simulink model "Uklad_Obiekt_Regulator_Calka150"  (R2024a)
settings: Solver=VariableStepAuto  StartTime=0.0  StopTime=10.0  RelTol=1e-3
values from neighbouring files (symbols this model uses):
  K = K_r(1:end-1)    [oblicz_parametry_obserwatora_z_calkowaniem.m]    (also in oblicz_parametry_regulatora.m = acker(A, B, [s_b s_b s_b]); symulacjeObserwator.m = oblicz_parametry_regulatora(A, B, s_b); symulacjeObserwatorZero.m = oblicz_parametry_regulatora(A, B, s_b); symulacjeRegulator.m = oblicz_parametry_regulatora(A, B, s_b))
  K_e = K_r(end)    [oblicz_parametry_obserwatora_z_calkowaniem.m]
  X_0 = [1; -5; 1]    [symulacjeObserwator.m]    (also in symulacjeObserwatorZero.m; symulacjeRegulator.m; symulacjeRegulatorCalka.m = [0; 0; 0]; symulacjeRegulatorCalka150.m = [0; 0; 0])
  y_zad = 10    [symulacjeRegulatorCalka.m]    (also in symulacjeRegulatorCalka150.m)
settings Model: Creator=pioro  LastModifiedBy=pioro

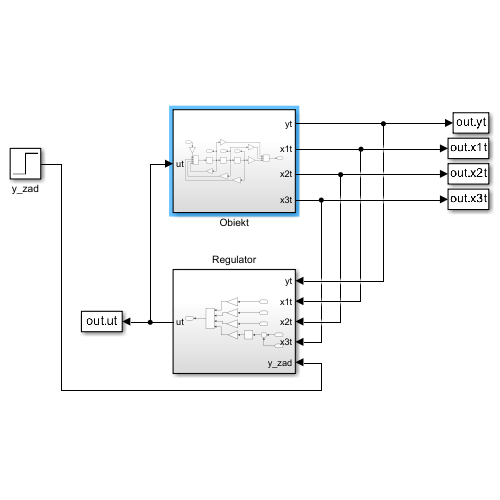
[thumbnail: Simulink's stored preview of the top-level diagram]
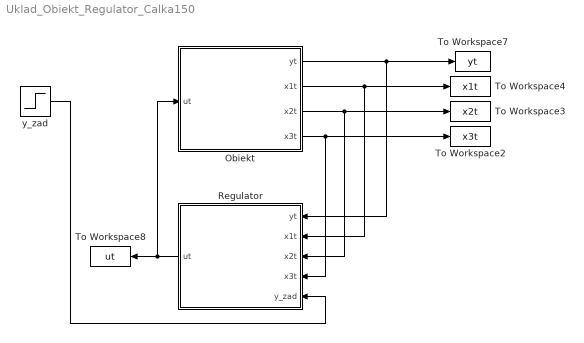
== system Uklad_Obiekt_Regulator_Calka150 ==
  Obiekt : Subsystem
  Regulator : Subsystem
  To Workspace2 : ToWorkspace  VariableName=x3t  SaveFormat=Timeseries  SampleTime=-1
  To Workspace3 : ToWorkspace  VariableName=x2t  SaveFormat=Timeseries  SampleTime=-1
  To Workspace4 : ToWorkspace  VariableName=x1t  SaveFormat=Timeseries  SampleTime=-1
  To Workspace7 : ToWorkspace  VariableName=yt  SaveFormat=Timeseries  SampleTime=-1
  To Workspace8 : ToWorkspace  VariableName=ut  SaveFormat=Timeseries  SampleTime=-1
  y_zad : Step  After=y_zad  SampleTime=0
  wires:
  Obiekt/3(x2t) -> To Workspace3/1, Regulator/3(x2t)
  y_zad/1 -> Regulator/5(y_zad)
  Obiekt/1(yt) -> Regulator/1(yt), To Workspace7/1
  Regulator/1(ut) -> Obiekt/1(ut), To Workspace8/1
  Obiekt/4(x3t) -> To Workspace2/1, Regulator/4(x3t)
  Obiekt/2(x1t) -> To Workspace4/1, Regulator/2(x1t)

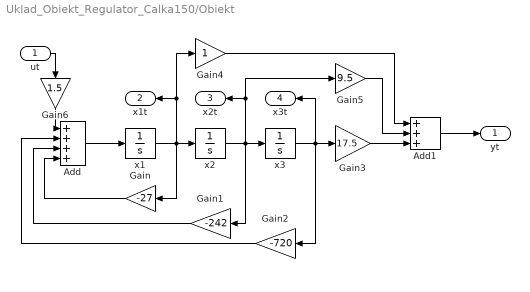
== system Uklad_Obiekt_Regulator_Calka150/Obiekt ==
  ut : Inport
  Add : Sum  Inputs=++++
  Add1 : Sum  Inputs=+++
  Gain : Gain  Gain=-27
  Gain1 : Gain  Gain=-242
  Gain2 : Gain  Gain=-720
  Gain3 : Gain  Gain=17.5
  Gain4 : Gain
  Gain5 : Gain  Gain=9.5
  Gain6 : Gain  Gain=1.5
  x1 : Integrator  InitialCondition=X_0(1)
  x2 : Integrator  InitialCondition=X_0(2)
  x3 : Integrator  InitialCondition=X_0(3)
  yt : Outport
  x1t : Outport  Port=2
  x2t : Outport  Port=3
  x3t : Outport  Port=4
  wires:
  x3/1 -> Gain2/1, Gain3/1, x3t/1
  ut/1 -> Gain6/1
  Gain4/1 -> Add1/1
  x1/1 -> Gain4/1, x1t/1, x2/1, Gain/1
  Gain1/1 -> Add/3
  Gain3/1 -> Add1/3
  Gain5/1 -> Add1/2
  Add1/1 -> yt/1
  Add/1 -> x1/1
  Gain2/1 -> Add/2
  Gain/1 -> Add/4
  x2/1 -> Gain5/1, x2t/1, x3/1, Gain1/1
  Gain6/1 -> Add/1

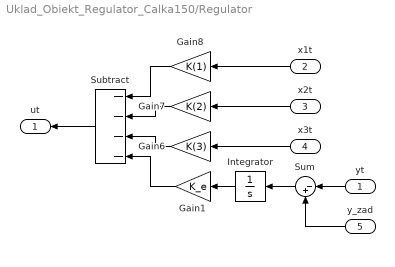
== system Uklad_Obiekt_Regulator_Calka150/Regulator ==
  yt : Inport
  x1t : Inport  Port=2
  x2t : Inport  Port=3
  x3t : Inport  Port=4
  y_zad : Inport  Port=5
  Gain1 : Gain  Gain=K_e
  Gain6 : Gain  Gain=K(3)
  Gain7 : Gain  Gain=K(2)
  Gain8 : Gain  Gain=K(1)
  Integrator : Integrator
  Subtract : Sum  Inputs=----
  Sum : Sum  Inputs=|-+
  ut : Outport
  wires:
  Gain7/1 -> Subtract/2
  Gain6/1 -> Subtract/3
  Gain8/1 -> Subtract/1
  x3t/1 -> Gain6/1
  Subtract/1 -> ut/1
  x1t/1 -> Gain8/1
  x2t/1 -> Gain7/1
  Integrator/1 -> Gain1/1
  Gain1/1 -> Subtract/4
  yt/1 -> Sum/1
  Sum/1 -> Integrator/1
  y_zad/1 -> Sum/2
